simulink model "cstr_sim"  (R2017b)
settings: Solver=ode45  StartTime=0.0  StopTime=10  RelTol=1e-3  EnableMultiTasking=on
StopFcn:
  | plot_reactor
libraries: simulink x5, realtime_pacer_lib x1
settings Model: Creator=tsladeche  LastModifiedBy=D A Santana
settings DataIOCC: LimitDataPoints=on  SaveFormat=Array  SignalLoggingSaveFormat=ModelDataLogs
settings OptimizationCC: ExpressionDepthLimit=2147483647  LifeSpan=inf
settings DebuggingCC: UnderspecifiedInitializationDetection=Classic  MergeDetectMultiDrivingBlocksExec=none  SolverPrmCheckMsg=warning  FcnCallInpInsideContextMsg=warning  StateNameClashWarn=warning  StrictBusMsg=Warning  SFUnexpectedBacktrackingDiag=warning  SFNoUnconditionalDefaultTransitionDiag=warning  SFExecutionAtInitializationDiag=none
settings HardwareCC: ProdBitPerPointer=32  ProdBitPerSizeT=32  ProdBitPerPtrDiffT=32  ProdLargestAtomicFloat=None  ProdIntDivRoundTo=Undefined  ProdEndianess=Unspecified  ProdWordSize=32  ProdHWDeviceType=32-bit Generic
settings ModelReferenceCC: PropagateSignalLabelsOutOfModel=off
settings CodeAppCC: StateflowObjectComments=on
settings GRTTargetCC: TargetLangStandard=C89/C90 (ANSI)  GeneratePreprocessorConditionals=Disable all  CombineOutputUpdateFcns=off  GRTInterface=on
settings ConfigComp: CovMetricSettings=dw  CovHtmlReporting=on  CovSaveCumulativeToWorkspaceVar=on  CovSaveSingleToWorkspaceVar=on  CovExternalEMLEnable=off

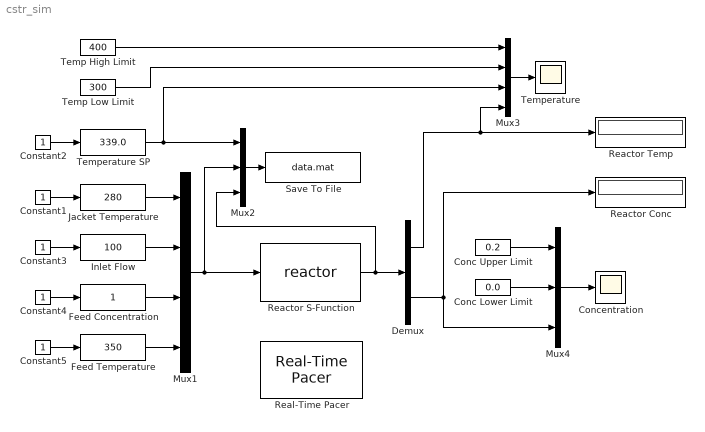
== system cstr_sim ==
  Conc Lower Limit : Constant  Value=0.0
  Conc Upper Limit : Constant  Value=0.2
  Concentration : Scope
  Constant{1..5} (5 alike) : Constant
  Demux : Demux  Outputs=2
  Feed Concentration : simulink/Math Operations/Slider Gain  gain=1  low=0  high=1
  Feed Temperature : simulink/Math Operations/Slider Gain  gain=350  low=300  high=400
  Inlet Flow : simulink/Math Operations/Slider Gain  gain=100  low=0  high=200
  Jacket Temperature : simulink/Math Operations/Slider Gain  gain=280  low=250  high=350
  Mux1 : Mux
  Mux2 : Mux  Inputs=3
  Mux3 : Mux
  Mux4 : Mux  Inputs=3
  Reactor Conc : Display
  Reactor S-Function : S-Function  FunctionName=reactor  SFunctionDeploymentMode=off  EnableBusSupport=off
  Reactor Temp : Display
  Real-Time Pacer : realtime_pacer_lib/Real-Time Pacer  simTimePerRealTime=1/5
  Save To File : ToFile  Filename=data.mat  MatrixName=cstr  SampleTime=0.05
  Temp High Limit : Constant  Value=400
  Temp Low Limit : Constant  Value=300
  Temperature : Scope
  Temperature SP : simulink/Math Operations/Slider Gain  gain=339.0  low=300  high=400
  wires:
  Reactor S-Function/1 -> Mux2/3, Demux/1
  Constant3/1 -> Inlet Flow/1
  Mux2/1 -> Save To File/1
  Constant1/1 -> Jacket Temperature/1
  Mux1/1 -> Mux2/2, Reactor S-Function/1
  Inlet Flow/1 -> Mux1/2
  Jacket Temperature/1 -> Mux1/1
  Constant2/1 -> Temperature SP/1
  Temperature SP/1 -> Mux3/3, Mux2/1
  Demux/2 -> Mux4/3, Reactor Conc/1
  Constant4/1 -> Feed Concentration/1
  Feed Concentration/1 -> Mux1/3
  Constant5/1 -> Feed Temperature/1
  Feed Temperature/1 -> Mux1/4
  Demux/1 -> Mux3/4, Reactor Temp/1
  Temp High Limit/1 -> Mux3/1
  Temp Low Limit/1 -> Mux3/2
  Mux3/1 -> Temperature/1
  Conc Upper Limit/1 -> Mux4/1
  Conc Lower Limit/1 -> Mux4/2
  Mux4/1 -> Concentration/1
